simulink model "sldemo_varsize_dataLengthAdapt_org"  (Simulink 10.0)
settings: Solver=FixedStepDiscrete  StartTime=0.0  StopTime=2.0  RelTol=1e-3  EnableMultiTasking=on
libraries: simulink x3
settings Model: Creator=The MathWorks, Inc.  LastModifiedBy=bhisma
settings DataIOCC: LimitDataPoints=on  SaveFormat=StructureWithTime  ReturnWorkspaceOutputs=on
settings OptimizationCC: ExpressionDepthLimit=2147483647
settings DebuggingCC: UnderspecifiedInitializationDetection=Simplified  MergeDetectMultiDrivingBlocksExec=error  SolverPrmCheckMsg=warning  FcnCallInpInsideContextMsg=warning  AllowSymbolicDim=off  StateNameClashWarn=warning
settings SFSimCC: SimParseCustomCode=off
settings GRTTargetCC: GeneratePreprocessorConditionals=Disable all
settings ConfigComp: CovExternalEMLEnable=off

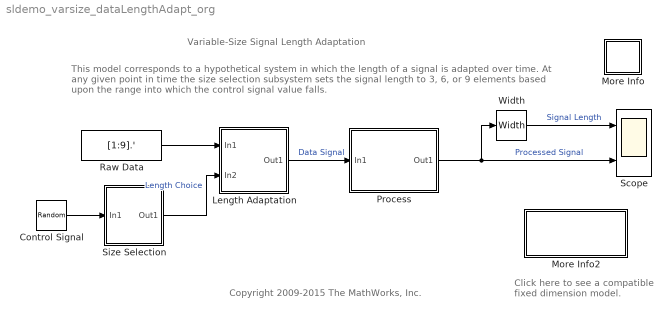
== system sldemo_varsize_dataLengthAdapt_org ==
  note: Variable-Size Signal Length Adaptation
  note: Copyright 2009-2015 The MathWorks, Inc.
  note: This model corresponds to a  hypothetical system in which the length of a signal is adapted over time.
      | At any given  point in time the size selection subsystem sets the signal length to 3, 6, or 9  elements based upon
      | the range into which the control signal value falls.
  note: Click here to see a compatible
      | fixed dimension model.
  Control Signal : RandomNumber  Variance=0.5  SampleTime=0.1
  Length Adaptation : Subsystem
  More Info : Subsystem
      settings: OpenFcn=showdemo(bdroot(gcb))
      mask Display: disp('?')
  More Info2 : Subsystem
      settings: OpenFcn=sldemo_varsize_dataLengthAdaptFixSizeImpl
      mask Display: disp('Fixed-Size Signal\nImplementation')
  Process : Subsystem
  Raw Data : Constant  Value=[1:9].'
  Scope : Scope  NumInputPorts=2
  Size Selection : Subsystem
  Width : Width
  wires:
  Length Adaptation/1(Out1) -> Process/1(In1)  "Data Signal"
  Width/1 -> Scope/1  "Signal Length"
  Size Selection/1(Out1) -> Length Adaptation/2(In2)  "Length Choice"
  Raw Data/1 -> Length Adaptation/1(In1)
  Process/1(Out1) -> Scope/2, Width/1  "Processed Signal"
  Control Signal/1 -> Size Selection/1(In1)

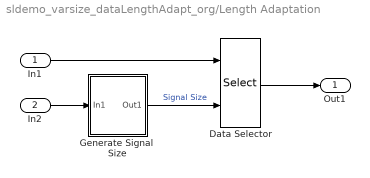
== system sldemo_varsize_dataLengthAdapt_org/Length Adaptation ==
  In1 : Inport
  In2 : Inport  Port=2
  Data Selector : Selector  InputPortWidth=9  IndexOptions=Starting and ending indices (port)  Indices=[1 3]  OutputSizes=32
  Generate Signal  Size : Subsystem
  Out1 : Outport  VectorParamsAs1DForOutWhenUnconnected=off
  wires:
  Data Selector/1 -> Out1/1
  In1/1 -> Data Selector/1
  In2/1 -> Generate Signal  Size/1(In1)
  Generate Signal  Size/1(Out1) -> Data Selector/2  "Signal Size"

== system sldemo_varsize_dataLengthAdapt_org/More Info ==
  note: Bus Block Demonstration
  note: This demonstration shows how signals may be grouped and ungrouped while
      | retaining their names.  In this demonstration, 5 signals are created and labelled
      | appropriately.  These signals are then muxed together to create a bus of signals.
      | This bus of signals is then fed into the Bus Selector block.  Inside of the Bus
      | Selector block, the Pulse and Chirp signals are chosen to be output from the
      | original signal bus.
      |
      | It is possible to place a nest signal buses and then still retrieve the original signal
      | with its label.

== system sldemo_varsize_dataLengthAdapt_org/More Info2 ==

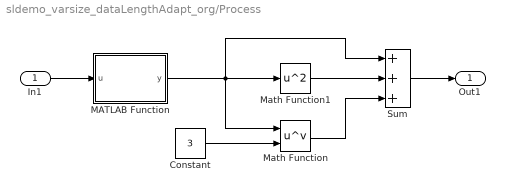
== system sldemo_varsize_dataLengthAdapt_org/Process ==
  In1 : Inport
      settings: VarSizeSig=Yes
  Constant : Constant  Value=3
  MATLAB Function : MATLAB Function  TreatAsAtomicUnit=on
  Math Function : Math  Operator=pow  SaturateOnIntegerOverflow=on
  Math Function1 : Math  Operator=square  SaturateOnIntegerOverflow=on
  Sum : Sum  Inputs=+++
  Out1 : Outport  VectorParamsAs1DForOutWhenUnconnected=off
  wires:
  In1/1 -> MATLAB Function/1(u)
  MATLAB Function/1(y) -> Math Function/1, Math Function1/1, Sum/1
  Math Function1/1 -> Sum/2
  Sum/1 -> Out1/1
  Constant/1 -> Math Function/2
  Math Function/1 -> Sum/3

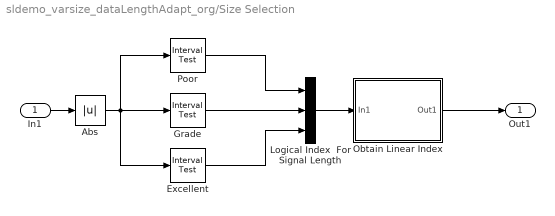
== system sldemo_varsize_dataLengthAdapt_org/Size Selection ==
  In1 : Inport
  Abs : Abs
  Excellent : simulink/Logic and Bit Operations/Interval Test  IntervalClosedRight=off  uplimit=inf  IntervalClosedLeft=on  lowlimit=0.50  OutDataTypeStr=uint8
  Grade : simulink/Logic and Bit Operations/Interval Test  IntervalClosedRight=off  uplimit=0.50  IntervalClosedLeft=on  lowlimit=0.25  OutDataTypeStr=uint8
  Logical Index  For Signal Length : Concatenate  NumInputs=3
  Obtain Linear Index : Subsystem
  Poor : simulink/Logic and Bit Operations/Interval Test  IntervalClosedRight=off  uplimit=0.25  IntervalClosedLeft=on  lowlimit=0.0  OutDataTypeStr=uint8
  Out1 : Outport  VectorParamsAs1DForOutWhenUnconnected=off
  wires:
  Obtain Linear Index/1(Out1) -> Out1/1
  Grade/1 -> Logical Index  For Signal Length/2
  Excellent/1 -> Logical Index  For Signal Length/3
  Poor/1 -> Logical Index  For Signal Length/1
  Logical Index  For Signal Length/1 -> Obtain Linear Index/1(In1)
  Abs/1 -> Grade/1, Poor/1, Excellent/1
  In1/1 -> Abs/1

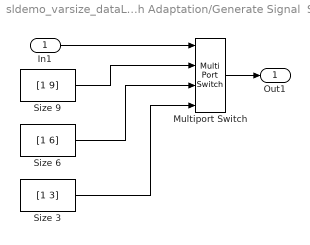
== system sldemo_varsize_dataLengthAdapt_org/Length Adaptation/Generate Signal  Size ==
  In1 : Inport
  Multiport Switch : MultiPortSwitch
  Size 3 : Constant  Value=[1 3]
  Size 6 : Constant  Value=[1 6]
  Size 9 : Constant  Value=[1 9]
  Out1 : Outport  VectorParamsAs1DForOutWhenUnconnected=off
  wires:
  Size 3/1 -> Multiport Switch/4
  Size 6/1 -> Multiport Switch/3
  Size 9/1 -> Multiport Switch/2
  In1/1 -> Multiport Switch/1
  Multiport Switch/1 -> Out1/1

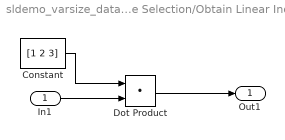
== system sldemo_varsize_dataLengthAdapt_org/Size Selection/Obtain Linear Index ==
  In1 : Inport
  Constant : Constant  Value=[1 2 3]
  Dot Product : DotProduct  OutDataTypeStr=Inherit: Inherit via internal rule
  Out1 : Outport  VectorParamsAs1DForOutWhenUnconnected=off
  wires:
  In1/1 -> Dot Product/2
  Dot Product/1 -> Out1/1
  Constant/1 -> Dot Product/1

== matlab function Process/MATLAB Function ==
  data: u input double size=9; y output double size=18
function y = fcn(u)
%#codegen
%
% Insert zeros between elements

sizeU = length(u);
y     = zeros(2*sizeU,1);
for i=1:2*sizeU
    if(mod(i,2))
        y(i)=0; 
    else
        y(i)=u(i/2)/10;
    end
end
